simulink model "WaveStar"  (R2024b)
settings: Solver=ode8  StartTime=0  StopTime=75  FixedStep=0.05  MaxStep=0.05  RelTol=1e-3  EnableMultiTasking=on
values from neighbouring files (symbols this model uses):
  Ad = sysD.A    [controller_init.m]
  alpha_eff = ( eta_motoring + eta_generator ) / 2    (= 1.06428571429)    [controller_init.m]
  ARorder = 18    [controller_init.m]
  ARtrainingSet = 10    [controller_init.m]
  Bd = sysD.B    [controller_init.m]
  beta_eff = ( eta_motoring - eta_generator ) / 2    (= 0.364285714286)    [controller_init.m]
  dt = simu.dt    [controller_init.m]
  eta_generator = 0.7    [controller_init.m]
  eta_motoring = 1 / 0.7    (= 1.42857142857)    [controller_init.m]
  excM_precalculated = excM_stored    [controller_init.m]
  L_AB = 0.412    [controller_init.m]
  L_AC = 0.2    [controller_init.m]
  LAfloat = 0.54875    [controller_init.m]
  McSat = 12    [controller_init.m]
  N = K_init:step:k_end    [MRC_K_prop.m]
  Np = 40    [controller_init.m]
  phi_eff = 1000    [controller_init.m]
  predictionType = 1    [controller_init.m]
  prop_gain = i    [MCR_K_prop.m]    (also in MRC_K_prop.m = N(run_ind); controller_init.m = 6.20;   load('waveData/SS4_excM_stored.mat'))
  Qkf = blkdiag( Qp, Qv, QradM, QexcM )    [controller_init.m]
  qnl = [ 0, 1; 1, 0 ]    [controller_init.m]
  R_ctrl = 0.90*eye( Np*nu )    [controller_init.m]
  Rkf = blkdiag( Rp, Rv )    [controller_init.m]
  simu = simulationClass()    [wecSimInputFile.m]
  startController = 15    [controller_init.m]
  startPredictor = 10    [controller_init.m]
  Theta0 = deg2rad(26.9527)    [controller_init.m]
  Umax = McSat    (= 12)    [controller_init.m]
  Umin = -McSat    (= -12)    [controller_init.m]
  waves = waveClass('irregular')    [wecSimInputFile.m]
  xPcTs = dt    [controller_init.m]
undefined symbols (not defined in the file or in its folder): body, constraint, HPfreq, hydroData, LPfreq, pto, X, Y, Z
libraries: nesl_utility x31, sm_lib x21, WECSim_Lib_Body_Elements x10, WECSim_Lib_Constraints x5, WECSim_Lib_Frames x1, vrlib x1
(part 4 of 4)

== system WaveStar/Rigid Body/Hydrodynamic Body/Morison Element and Viscous Damping Force Calculation/Morison Element Variant Subsystem/Morison Element On/No Wave Morison Force ==
  displacement : Inport
  velocity : Inport  Port=2
  acceleration : Inport  Port=3
  time : Inport  Port=4
  Area : Constant  Value=body.morisonElement.area  VectorParams1D=off
  Ca : Constant  Value=body.morisonElement.ca  VectorParams1D=off
  Cd : Constant  Value=body.morisonElement.cd  VectorParams1D=off
  Current Depth : Constant  Value=waves.current.depth
  Current Direction : Constant  Value=waves.current.direction
  Current Option : Constant  Value=waves.current.option
  Current Speed : Constant  Value=waves.current.speed
  Density : Constant  Value=simu.rho
  Morison Element Option : Constant  Value=body.morisonElement.option
  MorisonElement(s) : MATLAB Function  TreatAsAtomicUnit=on
  Ramp Function Time : Constant  Value=simu.rampTime
  Volume : Constant  Value=body.morisonElement.VME  VectorParams1D=off
  "r_{g}" : Constant  Value=body.morisonElement.rgME  VectorParams1D=off
  z : Constant  Value=body.morisonElement.z  VectorParams1D=off
  morison_force : Outport
  wires:
  MorisonElement(s)/1(f) -> morison_force/1
  z/1 -> MorisonElement(s)/1(z)
  "r_{g}"/1 -> MorisonElement(s)/2(r)
  velocity/1 -> MorisonElement(s)/3(Vel)
  acceleration/1 -> MorisonElement(s)/4(Accel)
  displacement/1 -> MorisonElement(s)/5(Disp)
  Area/1 -> MorisonElement(s)/6(Area)
  Cd/1 -> MorisonElement(s)/7(Cd)
  Volume/1 -> MorisonElement(s)/8(Vol)
  Ca/1 -> MorisonElement(s)/9(Ca)
  time/1 -> MorisonElement(s)/10(Time)
  Density/1 -> MorisonElement(s)/11(rho)
  Ramp Function Time/1 -> MorisonElement(s)/12(rampTime)
  Current Speed/1 -> MorisonElement(s)/13(currentSpeed)
  Current Direction/1 -> MorisonElement(s)/14(currentDirection)
  Current Depth/1 -> MorisonElement(s)/15(currentDepth)
  Current Option/1 -> MorisonElement(s)/16(currentOption)
  Morison Element Option/1 -> MorisonElement(s)/17(bodyMorison)

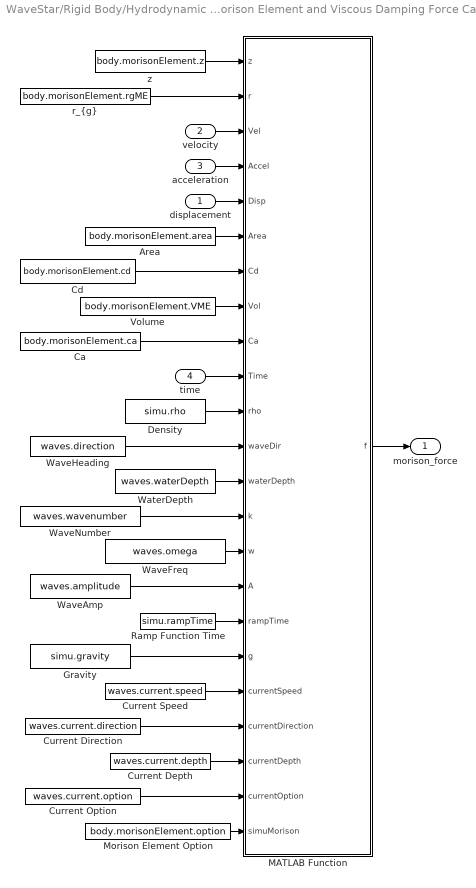
== system WaveStar/Rigid Body/Hydrodynamic Body/Morison Element and Viscous Damping Force Calculation/Morison Element Variant Subsystem/Morison Element On/Regular Wave Morison Force ==
  displacement : Inport
  velocity : Inport  Port=2
  acceleration : Inport  Port=3
  time : Inport  Port=4
  Area : Constant  Value=body.morisonElement.area  VectorParams1D=off
  Ca : Constant  Value=body.morisonElement.ca  VectorParams1D=off
  Cd : Constant  Value=body.morisonElement.cd  VectorParams1D=off
  Current Depth : Constant  Value=waves.current.depth
  Current Direction : Constant  Value=waves.current.direction
  Current Option : Constant  Value=waves.current.option
  Current Speed : Constant  Value=waves.current.speed
  Density : Constant  Value=simu.rho
  Gravity : Constant  Value=simu.gravity
  MATLAB Function : MATLAB Function  TreatAsAtomicUnit=on
  Morison Element Option : Constant  Value=body.morisonElement.option
  Ramp Function Time : Constant  Value=simu.rampTime
  Volume : Constant  Value=body.morisonElement.VME  VectorParams1D=off
  WaterDepth : Constant  Value=waves.waterDepth
  WaveAmp : Constant  Value=waves.amplitude
  WaveFreq : Constant  Value=waves.omega
  WaveHeading : Constant  Value=waves.direction
  WaveNumber : Constant  Value=waves.wavenumber
  "r_{g}" : Constant  Value=body.morisonElement.rgME  VectorParams1D=off
  z : Constant  Value=body.morisonElement.z  VectorParams1D=off
  morison_force : Outport
  wires:
  MATLAB Function/1(f) -> morison_force/1
  z/1 -> MATLAB Function/1(z)
  Morison Element Option/1 -> MATLAB Function/23(simuMorison)
  Volume/1 -> MATLAB Function/8(Vol)
  velocity/1 -> MATLAB Function/3(Vel)
  Ramp Function Time/1 -> MATLAB Function/17(rampTime)
  "r_{g}"/1 -> MATLAB Function/2(r)
  time/1 -> MATLAB Function/10(Time)
  Current Depth/1 -> MATLAB Function/21(currentDepth)
  Current Option/1 -> MATLAB Function/22(currentOption)
  displacement/1 -> MATLAB Function/5(Disp)
  Cd/1 -> MATLAB Function/7(Cd)
  WaveFreq/1 -> MATLAB Function/15(w)
  WaveHeading/1 -> MATLAB Function/12(waveDir)
  Density/1 -> MATLAB Function/11(rho)
  acceleration/1 -> MATLAB Function/4(Accel)
  WaterDepth/1 -> MATLAB Function/13(waterDepth)
  Area/1 -> MATLAB Function/6(Area)
  Current Direction/1 -> MATLAB Function/20(currentDirection)
  Ca/1 -> MATLAB Function/9(Ca)
  WaveNumber/1 -> MATLAB Function/14(k)
  Gravity/1 -> MATLAB Function/18(g)
  WaveAmp/1 -> MATLAB Function/16(A)
  Current Speed/1 -> MATLAB Function/19(currentSpeed)

== system WaveStar/Rigid Body/Hydrodynamic Body/Wave Radiation Forces Calculation/SS CI and Constant-Damping-CoeVariant Subsystem/FIR Filter Calculation/FIR Filter Matrix ==
  velocity : Inport
  FIR_filter_row : Subsystem  mask{body=body, B2B=simu.b2b, rowNo=1}
      mask prompts: body "BodyClass"
      mask init:
      | cb = gcb;
      | % The implementation that follows, calculates the radiation force, Fr, by
      | % calculating the Fr for each body mode by multiplying the velocity vector
      | % to the IRF matrix -- whose each row corresponds to the Fr for each of the
      | % modes corresponding to the velocity vector.
      | 
      | 
      | % Get the radiation IRF coefficients using body.hydroForce.irkb
      | set_param([cb '/Discrete FIR Filter'],...
      |            'position',[100, 0, 140, 180]);
      |          if rem(rowNo,6) ~= 0
      |         set_param([cb,'/Discrete FIR Filter'],...
      |                   'Coefficients', [sprintf('transpose(squeeze(body.hydroForce.hf1.irkb(:,%d,%d)))',rem(rowNo,6),1)]); 
      |          elseif rem(rowNo,6) == 0
      |         set_param([cb,'/Discrete FIR Filter'],...
      |                   'Coefficients', [sprintf('transpose(squeeze(body.hydroForce.hf1.irkb(:,%d,%d)))',6,1)]); 
      |          end
      | % Assign number of filters. The number of filter corresponds to the IRF
      | % matrix elements being used for the calculation for each row.
      | nFilt = body.dof + B2B*(body.total-1)*6;
      | 
      | % Add Demux channels corresponding to number of filters, and connect them to the corresponding filter.
      | 
      | set_param([cb '/Demux'],...
      |            'Outputs',sprintf('%d',nFilt));
      | try
      | add_line(cb,...
      |         'Demux/1',...
      |         ['Discrete FIR Filter','/1'], ...     
      |         'autorouting','on');
      | catch
      | end
      | 
      | try
      | add_line(cb,...
      |         'Discrete FIR Filter/1', ...     
      |         'Add/1',...
      |         'autorouting','on');
      | catch 
      | end
      | 
      | % Add filters 
      | 
      | for i = 2:nFilt
      | 
      |      try
      |         add_block([cb,'/Discrete FIR Filter'],[cb,'/Discrete FIR Filter ',num2str(i)],'MakeNameUnique','off',...
      |                    'Position',[100*i, 0, 40+100*i, 180],'BackgroundColor','white');
      |         signlist = get_param([cb,'/Add'],'Inputs');
      |         set_param([cb,'/Add'],'Inputs',[signlist,'+']);
      |      catch 
      |      end
      | 
      | 
      |      try
      |          if rem(rowNo,6) ~= 0
      |         set_param([cb,'/Discrete FIR Filter ',num2str(i)],...
      |                   'Coefficients', [sprintf('transpose(squeeze(body.hydroForce.hf1.irkb(:,%d,%d)))',rem(rowNo,6),i)]); 
      |          elseif rem(rowNo,6) == 0
      |         set_param([cb,'/Discrete FIR Filter ',num2str(i)],...
      |                   'Coefficients', [sprintf('transpose(squeeze(body.hydroForce.hf1.irkb(:,%d,%d)))',6,i)]); 
      |          end
      |      catch
      |      end
      | 
      |      try
      |         add_line(cb,...
      |         ['Demux/',num2str(i)],...
      |         ['Discrete FIR Filter ',num2str(i),'/1'], ...     
      |         'autorouting','on');
      |      catch
      |      end
      | 
      | 
      |      try
      |         add_line(cb,...
      |         ['Discrete FIR Filter ',num2str(i),'/1'], ...     
      |         ['Add/', num2str(i)],...
      |         'autorouting','on');
      |     catch 
      |     end
      | end
  Gain : Gain  Gain=simu.cicDt
  Mux : Mux  Inputs=1
  Out1 : Outport
  wires:
  Mux/1 -> Gain/1
  velocity/1 -> FIR_filter_row/1(In1)
  FIR_filter_row/1(Out1) -> Mux/1
  Gain/1 -> Out1/1

== system WaveStar/Rigid Body/Hydrodynamic Body/Wave Radiation Forces Calculation/SS CI and Constant-Damping-CoeVariant Subsystem/FIR Filter Calculation/FIR Filter Matrix/FIR_filter_row ==
  In1 : Inport
  Add : Sum  Inputs=++++++
  Demux : Demux  Outputs=6
      settings: AttributesFormatString=%<Outputs>
  Discrete FIR Filter : DiscreteFir  Coefficients=transpose(squeeze(body.hydroForce.hf1.irkb(:,1,1)))
  Discrete FIR Filter 2 : DiscreteFir  Coefficients=transpose(squeeze(body.hydroForce.hf1.irkb(:,1,2)))
  Discrete FIR Filter 3 : DiscreteFir  Coefficients=transpose(squeeze(body.hydroForce.hf1.irkb(:,1,3)))
  Discrete FIR Filter 4 : DiscreteFir  Coefficients=transpose(squeeze(body.hydroForce.hf1.irkb(:,1,4)))
  Discrete FIR Filter 5 : DiscreteFir  Coefficients=transpose(squeeze(body.hydroForce.hf1.irkb(:,1,5)))
  Discrete FIR Filter 6 : DiscreteFir  Coefficients=transpose(squeeze(body.hydroForce.hf1.irkb(:,1,6)))
  Out1 : Outport
  wires:
  In1/1 -> Demux/1
  Add/1 -> Out1/1
  Demux/1 -> Discrete FIR Filter/1
  Discrete FIR Filter/1 -> Add/1
  Demux/2 -> Discrete FIR Filter 2/1
  Discrete FIR Filter 2/1 -> Add/2
  Demux/3 -> Discrete FIR Filter 3/1
  Discrete FIR Filter 3/1 -> Add/3
  Demux/4 -> Discrete FIR Filter 4/1
  Discrete FIR Filter 4/1 -> Add/4
  Demux/5 -> Discrete FIR Filter 5/1
  Discrete FIR Filter 5/1 -> Add/5
  Demux/6 -> Discrete FIR Filter 6/1
  Discrete FIR Filter 6/1 -> Add/6

== matlab function WaveStar/Rigid Body/Hydrodynamic Body/Morison Element and Viscous Damping Force Calculation/Morison Element Variant Subsystem/Morison Element On/Irregular Wave Morison Force/MATLAB Function ==
  data: z input; f output; r input; Vel input; Accel input; Disp input; Area input; Cd input; Vol input; Ca input; Time input; rho input; waveDir input; waveSpread input; waterDepth input; k input; w input; A input; rampTime input; g input; randPhase input; dw input; currentSpeed input; currentDirection input; currentDepth input; currentOption input; simuMorison input
function f = irregWaveMorison(z,r,Vel,Accel,Disp,Area,Cd,Vol,Ca,Time,rho,waveDir,waveSpread,waterDepth,k,w,A,rampTime,g,randPhase,dw,currentSpeed,currentDirection,currentDepth,currentOption,simuMorison)

f = irregWaveMorison(z,r,Vel,Accel,Disp,Area,Cd,Vol,Ca,Time,rho,waveDir,waveSpread,waterDepth,k,w,A,rampTime,g,randPhase,dw,currentSpeed,currentDirection,currentDepth,currentOption,simuMorison);

end

== matlab function WaveStar/Rigid Body/Hydrodynamic Body/Morison Element and Viscous Damping Force Calculation/Morison Element Variant Subsystem/Morison Element On/No Wave Morison Force/MorisonElement(s) ==
  data: z input; f output; r input; Vel input; Accel input; Disp input; Area input; Cd input; Vol input; Ca input; Time input; rho input; rampTime input; currentSpeed input; currentDirection input; currentDepth input; currentOption input; bodyMorison input
function f = noWaveMorison(z,r,Vel,Accel,Disp,Area,Cd,Vol,Ca,Time,rho,rampTime,currentSpeed,currentDirection,currentDepth,currentOption,bodyMorison)

f = noWaveMorison(z,r,Vel,Accel,Disp,Area,Cd,Vol,Ca,Time,rho,rampTime,currentSpeed,currentDirection,currentDepth,currentOption,bodyMorison);

end

== matlab function WaveStar/Rigid Body/Hydrodynamic Body/Nonlinear Wave Elevation/Linear or Instantaneous Free Surface/Instantaneous Water Free Surface/Instantaneous FS ==
  data: x input; center input; f output; cg input; AH input; w input; dw input; k input; typeNum input; t input; rampT input; phaseRand input; waveDir input
function f  = waveElevation(x,center,cg,AH,w,dw,k,typeNum,t,rampT,phaseRand,waveDir)

f  = waveElevation(x,center,cg,AH,w,dw,k,typeNum,t,rampT,phaseRand,waveDir);

end

== matlab function WaveStar/Rigid Body/Hydrodynamic Body/Structure/Motion Sensor/quaternion2EulXYZ ==
  data: Q input; E output
function E = quaternion2EulXYZ(Q)

E = quaternion2EulXYZ(Q);

end

== matlab function WaveStar/Controller/controller_rot/Estimation Excitation Moment  ==
  settings: updateMethod=DISCRETE
  data: pos input; vel input; input_cmd input; states output; Ad parameter; Bd parameter; Qkf parameter; Rkf parameter
function states = observer(pos, vel, input_cmd,  Ad, Bd, Qkf, Rkf)
                       
    u = [pos;
         vel];

states = observer_kf(input_cmd, u, Ad, Bd, Qkf, Rkf);

== matlab function WaveStar/Controller/controller_rot/Prediction Excitation Moment /Prediction from Autoregressive Model  ==
  settings: updateMethod=DISCRETE
  data: waveExc input size=1; Np parameter size=1; ARorder parameter size=1; time input size=1; startPredictor parameter size=1; excM_pred output size=[Np, 1]; ARtrainingSet parameter size=1; dt parameter; excM_precalculated parameter; predictionType parameter
function excM_pred =  vectorExcMpred(waveExc, Np, ARorder, time, startPredictor, ARtrainingSet, dt, excM_precalculated, predictionType)
    coder.extrinsic('predictor');

    persistent past_excM
    if isempty(past_excM)
        past_excM = zeros( ARtrainingSet*ARorder, 1 );
    end

    past_excM = [past_excM(2:end,1); waveExc];
    excM_pred   = zeros(Np,1);
   
    if time >= startPredictor
        switch(predictionType)
        % 1 to use the precalculated excM obtained from wecSim.
        % 2 to use the excM prediction from the AR algorithm.
            case 1
                  currentTime_index = uint64( time / dt );
                  excM_pred  = excM_precalculated(currentTime_index + 1 : currentTime_index + Np );
            case 2
                  excM_pred  = predictor(past_excM, ARorder, Np, time);
         end 
    end

== matlab function WaveStar/Controller/controller_rot/Control strategy/RTI - NMPC Algorithm ==
  settings: updateMethod=DISCRETE
  data: xk0 input; ptoM output size=1; excM_pred input size=[Np,1]; Ad parameter; Bd parameter; R_ctrl parameter; Np parameter size=1; alpha_eff parameter size=1; beta_eff parameter size=1; phi_eff parameter size=1; qnl parameter; Umax parameter size=1; Umin parameter size=1; currenttime input size=1; startController parameter size=1; prop_gain parameter size=1
function ptoM = RTI_NMPC(xk0, excM_pred, Ad, Bd, R_ctrl, Np, alpha_eff, beta_eff, phi_eff, qnl, Umax, Umin,currenttime, startController, prop_gain)
    coder.extrinsic('NMPC');
    %Augmented system to include the previous control input in the state vector
    A   = blkdiag( Ad, 0 );                          %Augmented State Transition Matrix
    Bw  = [ Bd;  0 ];                                %Augmented Wave Input Matrix
    Bu  = [ Bd;  1 ];                                %Augmented Input Matrix
    Ubar = zeros(Np,1);
    if (currenttime >= 10) && (currenttime < startController)
       ptoM = - prop_gain * xk0(2);
    elseif (currenttime >= startController)
       Ubar = NMPC( xk0, excM_pred, A, Bu, Bw, R_ctrl, Np, alpha_eff, beta_eff, phi_eff, qnl, Umax, Umin);
       ptoM = Ubar(1,1);
    else
        ptoM = 0;
    end
    

   if ptoM >= Umax
       ptoM = Umax;
   elseif ptoM <= Umin
       ptoM = Umin;
   end

== matlab function WaveStar/Rigid Body/Hydrodynamic Body/Wave Diffraction and Excitation Force Calculation/Linear Wave Excitation Force Variant Subsystem/Irregular Wave Excitation Force/MATLAB Function ==
  data: A input; Fext output; w input; fExtRE input; fExtIM input; phaseRand input; dw input; time input; WaveDir input; spread input; fExtMD input
function Fext = irregExcF(A,w,fExtRE,fExtIM,phaseRand,dw,time,WaveDir,spread,fExtMD)

Fext = irregExcF(A,w,fExtRE,fExtIM,phaseRand,dw,time,WaveDir,spread,fExtMD);

end

== matlab function WaveStar/Rigid Body/Hydrodynamic Body/Wave Diffraction and Excitation Force Calculation/Linear Wave Excitation Force Variant Subsystem/Irregular Wave Excitation Force/MATLAB Function2 ==
  data: disp input; dispPhase output; enable input; frequency input; wavenumber input; direction input
function dispPhase  = calcDispPhase(disp, enable, frequency, wavenumber, direction)
% initialize
dispPhase = zeros(length(frequency),length(direction));
% execute
dispPhase = calcDispPhase(disp, enable, direction, frequency, wavenumber);

end

== matlab function WaveStar/Rigid Body/Hydrodynamic Body/Wave Diffraction and Excitation Force Calculation/Linear Wave Excitation Force Variant Subsystem/Irregular Wave NonLinearYaw/MATLAB Function ==
  data: A input; w input; dofGRD input; dirGRD input; wGRD input; fEHRE input; fEHIM input; Fext output; fEHMD input; phaseRand input; dw input; time input; direction input; spread input; Disp input; intThresh input; prevYaw input; relYawLast output; prevCoeffMD input; prevCoeffRE input; prevCoeffIM input; coeffsLastMD output; coeffsLastRE output; coeffsLastIM output
function [Fext,relYawLast,coeffsLastMD,coeffsLastRE,coeffsLastIM] = irregnLYaw(A,w,dofGRD,dirGRD,wGRD,fEHRE,fEHIM, fEHMD, phaseRand,dw,time,direction,spread, Disp, intThresh, prevYaw, prevCoeffMD, prevCoeffRE, prevCoeffIM)

%initialize outputs
Fext = zeros(1,6);
relYawLast=0;
coeffsLastMD=zeros(length(w),6);
coeffsLastRE=zeros(length(w),6);
coeffsLastIM=zeros(length(w),6);

[Fext,relYawLast,coeffsLastMD,coeffsLastRE,coeffsLastIM] = irregnLYaw(A,w,dofGRD,dirGRD,wGRD,fEHRE,fEHIM, fEHMD, phaseRand,dw,time,direction,spread, Disp, intThresh, prevYaw, prevCoeffMD, prevCoeffRE, prevCoeffIM);

end

== matlab function WaveStar/Rigid Body/Hydrodynamic Body/Wave Diffraction and Excitation Force Calculation/Linear Wave Excitation Force Variant Subsystem/Regular Wave Excitation Force/MATLAB Function1 ==
  data: disp input; dispPhase output; enable input; frequency input; wavenumber input; direction input
function dispPhase  = calcDispPhase(disp, enable, frequency, wavenumber, direction)
% initialize
dispPhase = zeros(length(frequency),length(direction));
% execute
dispPhase = calcDispPhase(disp, enable, direction, frequency, wavenumber);

end

== matlab function WaveStar/Rigid Body/Hydrodynamic Body/Wave Diffraction and Excitation Force Calculation/Linear Wave Excitation Force Variant Subsystem/Regular Wave NonLinear Yaw/MATLAB Function3 ==
  data: disp input; dispPhase output; enable input; frequency input; wavenumber input; direction input
function dispPhase  = calcDispPhase(disp, enable, frequency, wavenumber, direction)
% initialize
dispPhase = zeros(length(frequency),length(direction));
% execute
dispPhase = calcDispPhase(disp, enable, direction, frequency, wavenumber);

end

== matlab function WaveStar/Rigid Body/Hydrodynamic Body/Wave Diffraction and Excitation Force Calculation/Linear Wave Excitation Force Variant Subsystem/Regular Wave NonLinear Yaw/MATLAB Function1 ==
  data: A input; w input; dofGRD input; dirGRD input; fEHRE input; fEHIM input; Fext output; fEHMD input; time input; WaveDir input; Disp input; intThresh input; phase input; prevYaw input; relYawLast output; prevCoeffMD input; prevCoeffRE input; prevCoeffIM input; coeffsLastMD output; coeffsLastRE output; coeffsLastIM output
function [Fext,relYawLast,coeffsLastMD,coeffsLastRE,coeffsLastIM] = regnLYaw(A,w,dofGRD,dirGRD,fEHRE,fEHIM, fEHMD,time,WaveDir,Disp, intThresh, phase, prevYaw, prevCoeffMD, prevCoeffRE, prevCoeffIM)

%initialize outputs
Fext = zeros(1,6);
relYawLast=0;
coeffsLastMD=zeros(length(w),6); 
coeffsLastRE=zeros(length(w),6);
coeffsLastIM=zeros(length(w),6);

[Fext,relYawLast,coeffsLastMD,coeffsLastRE,coeffsLastIM] = regnLYaw(A,w,dofGRD,dirGRD,fEHRE,fEHIM, fEHMD,time,WaveDir,Disp, intThresh, phase, prevYaw, prevCoeffMD, prevCoeffRE, prevCoeffIM);

end

== matlab function WaveStar/Rigid Body/Hydrodynamic Body/Wave Diffraction and Excitation Force Calculation/Nonlinear FK Force Variant Subsystem/With Nonlinear FroudeKrylov Force/Diffraction and Excitation Forces ==
  data: x input; elv input; direction input; center input; f output; tnorm input; area input; rho input; g input; cg input; AH input; w input; dw input; wDepth input; deepWater input; k input; typeNum input; t input; phaseRand input; wp output; wpMeanFS output
function [f, wp, wpMeanFS]  = nonFKForce(x,elv,direction,center,tnorm,area,rho,g,cg,AH,w,dw,wDepth,deepWater,k,typeNum,t,phaseRand)

[f, wp, wpMeanFS]  = nonFKForce(x,elv,direction,center,tnorm,area,rho,g,cg,AH,w,dw,wDepth,deepWater,k,typeNum,t,phaseRand);

end

== matlab function WaveStar/Controller/controller_rot/Compute extracted Energy-Power ==
  data: vel input; P output; tor input; E output; eta_generator parameter; eta_motoring parameter; dt parameter
function [P, E] = Power(vel,tor, eta_generator, eta_motoring, dt)
                
    [P, E] = extractedPower(vel,tor, eta_generator, eta_motoring, dt);

== matlab function WaveStar/Rigid Body/Hydrodynamic Body/Wave Diffraction and Excitation Force Calculation/Second Order Excitation Force Variant Subsystem/With Second Order Excitation Force/Diffraction and Excitation Forces ==
  data: time_vector input; fastVaryingForce input; f output; slowVaryingForce input; t input
function f   = secondOrderExt(time_vector,fastVaryingForce,slowVaryingForce,t)

f  = secondOrderExt(time_vector,fastVaryingForce,slowVaryingForce,t);

end

== matlab function WaveStar/Rigid Body/Hydrodynamic Body/Wave Radiation Forces Calculation/SS CI and Constant-Damping-CoeVariant Subsystem/Convolution Integral Calculation/MATLAB Function1 ==
  data: velocity input; F_FM output; IRKB input; cicTime input
function F_FM = ConvolutionIntegral_interp(velocity, IRKB, cicTime)

F_FM = ConvolutionIntegral_interp(velocity, IRKB, cicTime);

end

== matlab function WaveStar/Rigid Body/Hydrodynamic Body/Morison Element and Viscous Damping Force Calculation/Morison Element Variant Subsystem/Morison Element On/Regular Wave Morison Force/MATLAB Function ==
  data: z input; f output; r input; Vel input; Accel input; Disp input; Area input; Cd input; Vol input; Ca input; Time input; rho input; waveDir input; waterDepth input; k input; w input; A input; rampTime input; g input; currentSpeed input; currentDirection input; currentDepth input; currentOption input; simuMorison input
function f = regWaveMorison(z,r,Vel,Accel,Disp,Area,Cd,Vol,Ca,Time,rho,waveDir,waterDepth,k,w,A,rampTime,g,currentSpeed,currentDirection,currentDepth,currentOption,simuMorison)

f = regWaveMorison(z,r,Vel,Accel,Disp,Area,Cd,Vol,Ca,Time,rho,waveDir,waterDepth,k,w,A,rampTime,g,currentSpeed,currentDirection,currentDepth,currentOption,simuMorison);

end

== matlab function WaveStar/Controller/controller_rot/Control strategy/Resistive Controller ==
  settings: updateMethod=DISCRETE
  data: xk0 input; ptoM output size=1; excM_pred input size=[Np,1]; Umax parameter size=1; Umin parameter size=1; currenttime input size=1; startController parameter size=1; prop_gain parameter size=1
function ptoM = resistive(xk0, excM_pred, Umax, Umin,currenttime, startController, prop_gain)

    if currenttime >= startController
       ptoM = - prop_gain * xk0(2);
           if ptoM >= Umax
               ptoM = Umax;
           elseif ptoM<=Umin
               ptoM = Umin;
           end
    else
        ptoM = 0*excM_pred(1);
    end

== matlab function WaveStar/Rigid Body/Hydrodynamic Body/Yaw Force Transforms/Yaw Force Transforms ==
  data: yaw input; F_Excitation output; dispGlobal input; F_RadiationDampingLocal input; F_AddedMassLocal input; F_ExcitationLocal input; F_RadiationDamping output; F_RestoringLocal input; F_AddedMass output; F_Restoring output
function [F_Excitation, F_RadiationDamping, F_AddedMass, F_Restoring] = fYawTransforms(yaw, dispGlobal, F_RadiationDampingLocal, F_AddedMassLocal, F_ExcitationLocal, F_RestoringLocal)

[F_Excitation, F_RadiationDamping, F_AddedMass, F_Restoring] = fYawTransforms(yaw, dispGlobal, F_RadiationDampingLocal, F_AddedMassLocal, F_ExcitationLocal, F_RestoringLocal);

end

== matlab function WaveStar/Rigid Body/Hydrodynamic Body/Yaw Kinematic Transforms/No B2B/Yaw Kinematic Transforms ==
  data: yaw input; dispLoc output; dispGlobal input; velGlobal input; accGlobal input; velLoc output; accLoc output
function [dispLoc, velLoc, accLoc] = kinYawTransform(yaw, dispGlobal, velGlobal, accGlobal)

[dispLoc, velLoc, accLoc] = kinYawTransformNoB2B(yaw, dispGlobal, velGlobal, accGlobal);

end

== matlab function WaveStar/Rigid Body/Hydrodynamic Body/Wave Diffraction and Excitation Force Calculation/Linear Wave Excitation Force Variant Subsystem/Irregular Wave NonLinearYaw/MATLAB Function1 ==
  data: disp input; dispPhase output; enable input; frequency input; wavenumber input; direction input
function dispPhase  = calcDispPhase(disp, enable, frequency, wavenumber, direction)
% initialize
dispPhase = zeros(length(frequency),length(direction));
% execute
dispPhase = calcDispPhase(disp, enable, direction, frequency, wavenumber);

end

== matlab function WaveStar/Rigid Body/Hydrodynamic Body/Yaw Kinematic Transforms/With B2B/Yaw Kinematic Transforms ==
  data: yaw input; dispLoc output; dispGlobal input; velGlobal input; accGlobal input; velLoc output; accLoc output; numBody parameter
function [dispLoc, velLoc, accLoc] = kinYawTransformB2B(yaw, dispGlobal, velGlobal, accGlobal, numBody)

[dispLoc, velLoc, accLoc] = kinYawTransformB2B(yaw, dispGlobal, velGlobal, accGlobal, numBody);

end

== matlab function WaveStar/Controller/lin2rot conversion/Linear2Angular Conversion/MATLAB Function1 K [m] ==
  data: u input; y output; L_AB parameter; L_AC parameter
function y = fcn(u,L_AB,L_AC)
%#codegen
y = L_AB'*L_AC'*sin(u);

== matlab function WaveStar/Controller/lin2rot conversion/Linear2Angular Conversion/MATLAB Function1 L_BC [m] ==
  data: u input; y output; L_BC_neutral parameter
 function y = fcn(u,L_BC_neutral)
%#codegen
%
y = u+L_BC_neutral';

== matlab function WaveStar/Controller/lin2rot conversion/Linear2Angular Conversion/MATLAB Function1 Theta [rad] ==
  data: u input; y output; a_CAB_neutral parameter
function y = fcn(u,a_CAB_neutral)
%#codegen
y = u-a_CAB_neutral';

== matlab function WaveStar/Controller/Transform excitation forces in excitation Moment around A ==
  data: u input; theta input size=1; y output size=1; LAfloat parameter size=1; Theta0 parameter size=1
function y = transfExcMoment( u, theta, LAfloat, Theta0)

xFexc       = u( 1 );
zFexc       = u( 3 );
pitchMexc   = u( 5 );

y = (-LAfloat * xFexc .*sin( Theta0 + theta ) - zFexc * LAfloat.*cos( Theta0 + theta ) + pitchMexc );

== matlab function WaveStar/Controller/lin2rot conversion/Linear2Angular Conversion/MATLAB Function1 a_CAB [rad] ==
  data: u input; y output; L_AB parameter; L_AC parameter
function y = fcn(u,L_AB,L_AC)
%#codegen
%
y = acos((u.^2-L_AB'^2-L_AC'^2)/(-2*L_AB'*L_AC'));

== matlab function WaveStar/Rigid Body/Hydrodynamic Body/Hydrostatic Restoring Force Calculation/Linear and Nonlinear Restoring Force Variant Subsystem/Nonlinear Hydrostatic Restoring Force/Restoring Forces ==
  data: x input; elv input; center input; f output; tnorm input; area input; rho input; g input; cg input; p output; mass input
function [f,p]  = nonLinearBuoyancy(x,elv,center,tnorm,area,rho,g,cg,mass)

[f,p]  = nonLinearBuoyancy(x,elv,center,tnorm,area,rho,g,cg,mass);

end
